simulink model "PWM_model_4screenshot"  (R2024b)
settings: Solver=odeN  StartTime=0.0  StopTime=35  MaxStep=5e-05  RelTol=0.001  EnableMultiTasking=on
InitFcn:
  | load bldcData
model workspace (MAT data in the model file):
  encoderResolution = 2000
  hallOffset = '0.5'
  indexOffset = 850
  polePairs = '4'
undefined symbols (not defined in the file or in its folder): Hecate_speed, Ts_motor
libraries: fl_lib x5, nesl_utility x2, ee_lib x1
settings Model: SimulationMode=accelerator  Creator=The MathWorks, Inc.  LastModifiedBy=andrea
settings SolverCC: ConsecutiveZCsStepRelTol=2.8421709430404e-13  AlgebraicLoopSolver=TrustRegion  AutoInsertRateTranBlk=on
settings DataIOCC: LimitDataPoints=on  SaveFormat=Array
settings OptimizationCC: DefaultParameterBehavior=Inlined  OptimizeBlockIOStorage=off  BufferReuse=off  GlobalBufferReuse=off  ExpressionFolding=off  ExpressionDepthLimit=2147483647  LocalBlockOutputs=off  ZeroExternalMemoryAtStartup=off  InitFltsAndDblsToZero=on  NoFixptDivByZeroProtection=on  EfficientFloat2IntCast=on  EfficientMapNaN2IntZero=off  LifeSpan=Inf  MaxStackSize=64  OptimizeDataStoreBuffers=off  BusAssignmentInplaceUpdate=off  EfficientTunableParamExpr=on
settings DebuggingCC: ReadBeforeWriteMsg=DisableAll  WriteAfterWriteMsg=DisableAll  WriteAfterReadMsg=DisableAll  CheckSSInitialOutputMsg=off  SignalResolutionControl=TryResolveAllWithWarning  SolverPrmCheckMsg=warning  InheritedTsInSrcMsg=none  MultiTaskDSMMsg=none  MultiTaskCondExecSysMsg=none  TasksWithSamePriorityMsg=none  SigSpecEnsureSampleTimeMsg=none  IntegerOverflowMsg=none  ParameterPrecisionLossMsg=none  FcnCallInpInsideContextMsg=warning  UnconnectedInputMsg=warning  UnconnectedOutputMsg=warning  UnconnectedLineMsg=warning  AllowSymbolicDim=off  StateNameClashWarn=warning  PregeneratedLibrarySubsystemCodeDiagnostic=none  SFUnexpectedBacktrackingDiag=warning  SFNoUnconditionalDefaultTransitionDiag=warning  SFExecutionAtInitializationDiag=none  IntegerSaturationMsg=none  ArithmeticOperatorsInVariantConditions=warning
settings HardwareCC: ProdBitPerChar=16  ProdBitPerInt=16  ProdBitPerPointer=32  ProdBitPerSizeT=32  ProdBitPerPtrDiffT=32  ProdLargestAtomicInteger=Integer  ProdLargestAtomicFloat=None  ProdWordSize=16  ProdLongLongMode=on  ProdHWDeviceType=Texas Instruments->C2000  TargetBitPerChar=16  TargetBitPerInt=16  TargetBitPerPointer=16  TargetLargestAtomicInteger=Integer  TargetIntDivRoundTo=Zero  TargetEndianess=LittleEndian  TargetWordSize=16  TargetHWDeviceType=TI C2000
settings ModelReferenceCC: EnableRefExpFcnMdlSchedulingChecks=on  PropagateSignalLabelsOutOfModel=off
settings SFSimCC: SimUseLocalCustomCode=off  MATLABDynamicMemAlloc=off
settings RTWCC: Description=Embedded Coder  SystemTargetFile=ert.tlc  TemplateMakefile=ert_default_tmf  GenerateReport=on  RTWUseLocalCustomCode=off  Toolchain=Texas Instruments Code Composer Studio (C2000)  IncludeHyperlinkInReport=on  LaunchReport=on  GenerateTraceInfo=on  GenerateTraceReport=on  GenerateTraceReportSl=on  GenerateTraceReportSf=on  GenerateTraceReportEml=on  GPUComputeCapability=3.5
settings CodeAppCC: IgnoreCustomStorageClasses=off  CustomSymbolStrType=$N$R$M  StateflowObjectComments=on  InternalIdentifier=Classic
settings ERTTargetCC: MultiwordLength=2048  InlinedParameterPlacement=Hierarchical  ERTCustomFileTemplate=example_file_process.tlc  ConvertIfToSwitch=off  SuppressUnreachableDefaultCases=off  MemSecPackage=tic2000demospkg  DynamicArrayContainerType=coder::array
settings ConfigComp: CovMetricSettings=dw  CovSaveCumulativeToWorkspaceVar=on  CovSaveSingleToWorkspaceVar=on  CovExternalEMLEnable=off  CovSFcnEnable=off

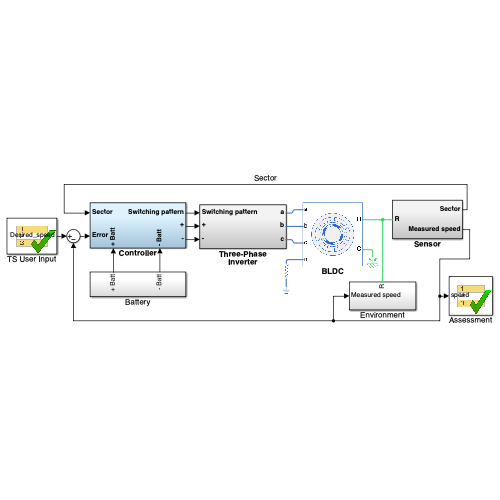
[thumbnail: Simulink's stored preview of the top-level diagram]
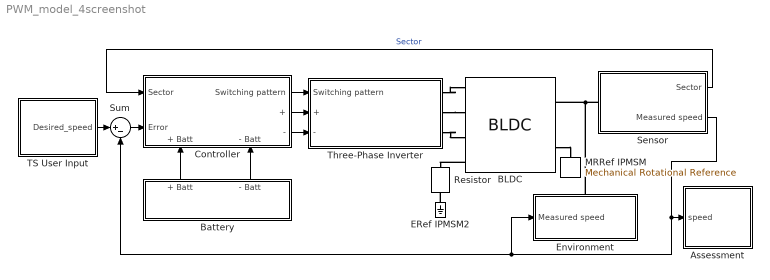
== system PWM_model_4screenshot ==
  Assessment : Test Sequence  TreatAsAtomicUnit=on
  BLDC : ee_lib/Electromechanical/Permanent Magnet/BLDC  port_option=ee.enum.threePhasePort.expanded  rotor_param=ee.enum.pmsm.backemf.trapezoidbackemf  pm_flux_linkage=0.18 Wb  theta_constant=120/23 deg  emf_max=20 V  w_meas=300 rpm  DphiDtheta_tab=[0, -.1528, -.1528, .1528, .1528, 0] Wb/rad  back_emf_tab=[0, -9.6, -9.6, 9.6, 9.6, 0] V  rotor_angle_tab=[0, 7.5, 22.5, 37.5, 52.5, 60] deg  nPolePairs=23  axes_param=ee.enum.rotorangle.daxis  winding_type=ee.enum.statorconnection.wye  stator_param=ee.enum.statorparam.LsLmMs  machine_param=ee.enum.dqparameterization.constant  Ld=0.00026 H  Lq=0.00026 H  idVec=[-200, 0, 200] A  iqVec=[-200, 0, 200] A  LdMatrix=0.00022 * ones(3, 3) H  LqMatrix=0.00022 * ones(3, 3) H  L0=0.00016 H  Ls=0.00026 H  Lm=0 H  Ms=0.00002 H  Rs=0.12 Ohm  zero_sequence=ee.enum.park.zerosequence.include  loss_param=ee.enum.ironloss.none  losses_oc=[0, 0, 0] W  losses_sc=[0, 0, 0] W  f_losses=60 Hz  Isc_losses=95 A  J=0 kg*m^2  lam=0.1 N*m/(rad/s)  i_d_specify=off  i_d_priority=None  i_d=0 A  i_d_nominal_specify=off  i_d_nominal_value=1  i_d_nominal_unit=A  i_q_specify=off  i_q_priority=None  i_q=0 A  i_q_nominal_specify=off  i_q_nominal_value=1  i_q_nominal_unit=A  torque_specify=off  torque_priority=None  torque=0 N*m  torque_nominal_specify=off  torque_nominal_value=1  torque_nominal_unit=N*m  angular_velocity_specify=off  angular_velocity_priority=High  angular_velocity=0 rpm  angular_velocity_nominal_specify=off  angular_velocity_nominal_value=1  angular_velocity_nominal_unit=rpm  angular_position_specify=off  angular_position_priority=High  angular_position=0 deg  angular_position_nominal_specify=off  angular_position_nominal_value=1  angular_position_nominal_unit=deg  alpha=3.93e-3 1/K  alpha_flux=-0.001 1/K  Tmeas=298.15 K  stator_thermal_mass=100 J/K  rotor_thermal_mass=200 J/K  Rm_percent_rotor=90  Rd_percent_rotor=30  temperatureA_specify=off  temperatureA_priority=High  temperatureA=25 degC  temperatureA_nominal_specify=off  temperatureA_nominal_value=1  temperatureA_nominal_unit=degC  temperatureB_specify=off  temperatureB_priority=High  temperatureB=25 degC  temperatureB_nominal_specify=off  temperatureB_nominal_value=1  temperatureB_nominal_unit=degC  temperatureC_specify=off  temperatureC_priority=High  temperatureC=25 degC  temperatureC_nominal_specify=off  temperatureC_nominal_value=1  temperatureC_nominal_unit=degC  temperatureR_specify=off  temperatureR_priority=High  temperatureR=25 degC  temperatureR_nominal_specify=off  temperatureR_nominal_value=1  temperatureR_nominal_unit=degC
      settings: InternalSimscapePortConfiguration="{\"Bottom\":[],\"Left\":[{\"id\":\"a\",\"label\":\"a\",\"type\":\"foundation.electrical.electrical\"},{\"id\":\"b\",\"label\":\"b\",\"type\":\"foundation.electrical.electrical\"},{\"id\":\"c\",\"label\":\"c\",\"type\":\"foundation.electrical.electrical\"},{\"id\":\"n\",\"label\":\"n\",\"type\":\"foundation.electrical.electrical\"}],\"Right\":[{\"id\":\"R\",\"label\":\"R\",\"type\":\"foundation.mechanical.rotational.rotational\"},{\"id\":\"C\",\"label\":\"C\",\"type\":\"foundation.mechanical.rotational.rotational\"}],\"Top\":[]}"
  Battery : Subsystem
      settings: PortSchema="{\"entries\":[{\"content\":{\"sides\":[{\"content\":{},\"type\":\"ConnectorPlacement.EquallySpacedRectSide\",\"uuid\":\"b9718aef-fc37-4786-bd99-1dccf9b07c4f\"},{\"content\":{\"side\":\"RIGHT\"},\"type\":\"ConnectorPlacement.EquallySpacedRectSide\",\"uuid\":\"5820c9b3-5480-4dfb-8619-e8171224d142\"},{\"content\":{\"connectorIds\":[\"Out1\",\"Out2\"],\"side\":\"TOP\"},\"type\":\"ConnectorPlacement.EquallySpacedRectSide\",\"uuid\":\"c449666b-5582-45da-b4a5-53b32c40c228\"}]},\"type\":\"ConnectorPlacement.EquallySpacedConnector\",\"uuid\":\"1a96bb2a-99ae-4235-9339-f0a559bfd98e\"}],\"packageUris\":[\"http://schema.mathworks.com/mf0/Connector/R2020b\"],\"version\":\"1.0\"}"
  Controller : Subsystem
      settings: PortSchema="{\"entries\":[{\"content\":{\"sides\":[{\"content\":{\"connectorIds\":[\"In1\",\"In2\"]},\"type\":\"ConnectorPlacement.EquallySpacedRectSide\",\"uuid\":\"2ab9d340-b50e-4422-9f4a-f0df7672da06\"},{\"content\":{\"connectorIds\":[\"Out1\",\"Out2\",\"Out3\"],\"side\":\"RIGHT\"},\"type\":\"ConnectorPlacement.EquallySpacedRectSide\",\"uuid\":\"8a4a8f23-4dad-4f8d-b073-fdebce0398f2\"},{\"content\":{\"side\":\"TOP\"},\"type\":\"ConnectorPlacement.EquallySpacedRectSide\",\"uuid\":\"b8c5a98d-225d-4655-b3bc-dd2e061911fb\"},{\"content\":{\"connectorIds\":[\"In3\",\"In4\"],\"side\":\"BOTTOM\"},\"type\":\"ConnectorPlacement.EquallySpacedRectSide\",\"uuid\":\"b2d3fee4-6eef-4d21-a73a-f8383ccb3ce8\"}]},\"type\":\"ConnectorPlacement.EquallySpacedConnector\",\"uuid\":\"adbcbcaa-ff3a-439a-b018-a3a47520a1df\"}],\"packageUris\":[\"http://schema.mathworks.com/mf0/Connector/R2020b\"],\"version\":\"1.0\"}"
  ERef IPMSM2 : fl_lib/Electrical/Electrical Elements/Electrical Reference
  Environment : Subsystem
      settings: PortSchema="{\"entries\":[{\"content\":{\"sides\":[{\"content\":{\"connectorIds\":[\"In1\"]},\"type\":\"ConnectorPlacement.EquallySpacedRectSide\",\"uuid\":\"b9718aef-fc37-4786-bd99-1dccf9b07c4f\"},{\"content\":{\"side\":\"RIGHT\"},\"type\":\"ConnectorPlacement.EquallySpacedRectSide\",\"uuid\":\"5820c9b3-5480-4dfb-8619-e8171224d142\"},{\"content\":{\"connectorIds\":[\"LConn1\"],\"side\":\"TOP\"},\"type\":\"ConnectorPlacement.EquallySpacedRectSide\",\"uuid\":\"c449666b-5582-45da-b4a5-53b32c40c228\"}]},\"type\":\"ConnectorPlacement.EquallySpacedConnector\",\"uuid\":\"1a96bb2a-99ae-4235-9339-f0a559bfd98e\"}],\"packageUris\":[\"http://schema.mathworks.com/mf0/Connector/R2020b\"],\"version\":\"1.0\"}"
  MRRef IPMSM : fl_lib/Mechanical/Rotational Elements/Mechanical Rotational Reference
  Resistor : fl_lib/Electrical/Electrical Elements/Resistor  R=1e9 Ohm  i_specify=off  i_priority=None  i=0 A  i_nominal_specify=off  i_nominal_value=1  i_nominal_unit=A  v_specify=off  v_priority=None  v=0 V  v_nominal_specify=off  v_nominal_value=1  v_nominal_unit=V
  Sensor : Subsystem
  Sum : Sum  Inputs=|+-
  TS User Input : Test Sequence  TreatAsAtomicUnit=on
  Three-Phase Inverter : Subsystem
  wires:
  Sensor/1(Sector) -> Controller/1(Sector)  "Sector"
  Sum/1 -> Controller/2(Error)
  TS User Input/1(Desired_speed) -> Sum/1
  Controller/1(Switching pattern) -> Three-Phase Inverter/1(Switching pattern)
  Battery/1(+ Batt) -> Controller/3(+ Batt)
  Battery/2(- Batt) -> Controller/4(- Batt)
  Controller/2(+) -> Three-Phase Inverter/2(+)
  Controller/3(-) -> Three-Phase Inverter/3(-)
  Sensor/2(Measured speed) -> Environment/1(Measured speed), Sum/2, Assessment/1(speed)
  connections:
  ERef IPMSM2/LConn1 -- Resistor/RConn1
  BLDC/LConn4 -- Resistor/LConn1
  Sensor/LConn1 -- Environment/LConn1 -- BLDC/RConn1
  BLDC/RConn2 -- MRRef IPMSM/LConn1
  Three-Phase Inverter/RConn1 -- BLDC/LConn1
  Three-Phase Inverter/RConn2 -- BLDC/LConn2
  Three-Phase Inverter/RConn3 -- BLDC/LConn3

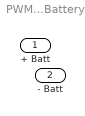
== system PWM_model_4screenshot/Battery ==
  + Batt : Outport
  - Batt : Outport  Port=2

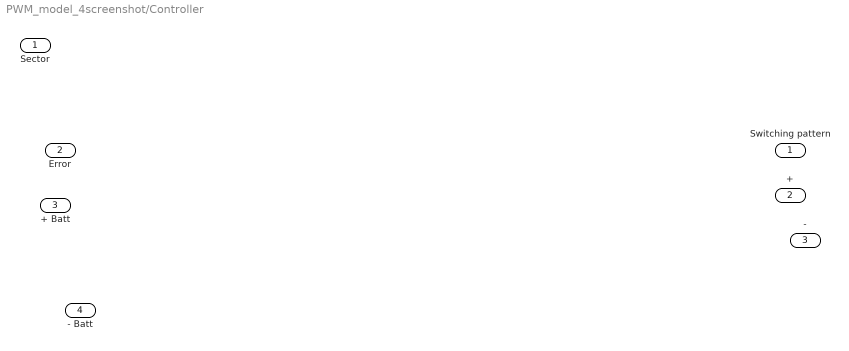
== system PWM_model_4screenshot/Controller ==
  Sector : Inport
  Error : Inport  Port=2
  + Batt : Inport  Port=3
  - Batt : Inport  Port=4
  Switching pattern : Outport
  + : Outport  Port=2
  - : Outport  Port=3

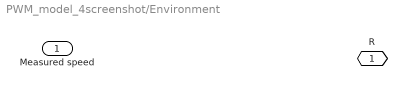
== system PWM_model_4screenshot/Environment ==
  Measured speed : Inport
  R : PMIOPort  Side=Left

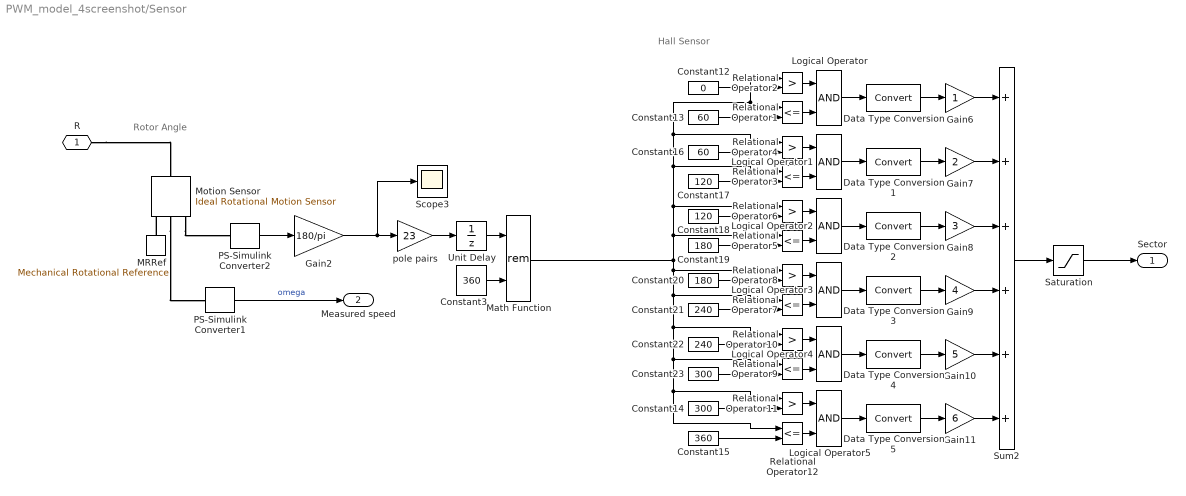
== system PWM_model_4screenshot/Sensor ==
  note: Rotor Angle
  note: Hall Sensor
  Constant12 : Constant  Value=0
  Constant13 : Constant  Value=60
  Constant14 : Constant  Value=300
  Constant15 : Constant  Value=360
  Constant16 : Constant  Value=60
  Constant17 : Constant  Value=120
  Constant18 : Constant  Value=120
  Constant19 : Constant  Value=180
  Constant20 : Constant  Value=180
  Constant21 : Constant  Value=240
  Constant22 : Constant  Value=240
  Constant23 : Constant  Value=300
  Constant3 : Constant  Value=360
  Data Type Conversion{,1..5} (6 alike) : DataTypeConversion
  Gain10 : Gain  Gain=5  SaturateOnIntegerOverflow=on  OutDataTypeStr=Inherit: Same as input  ParamDataTypeStr=Inherit: Same as input
  Gain11 : Gain  Gain=6  SaturateOnIntegerOverflow=on  OutDataTypeStr=Inherit: Same as input  ParamDataTypeStr=Inherit: Same as input
  Gain2 : Gain  Gain=180/pi
  Gain6 : Gain  SaturateOnIntegerOverflow=on  OutDataTypeStr=Inherit: Same as input  ParamDataTypeStr=Inherit: Same as input
  Gain7 : Gain  Gain=2  SaturateOnIntegerOverflow=on  OutDataTypeStr=Inherit: Same as input  ParamDataTypeStr=Inherit: Same as input
  Gain8 : Gain  Gain=3  SaturateOnIntegerOverflow=on  OutDataTypeStr=Inherit: Same as input  ParamDataTypeStr=Inherit: Same as input
  Gain9 : Gain  Gain=4  SaturateOnIntegerOverflow=on  OutDataTypeStr=Inherit: Same as input  ParamDataTypeStr=Inherit: Same as input
  Logical Operator{,1..5} (6 alike) : Logic
  MRRef : fl_lib/Mechanical/Rotational Elements/Mechanical Rotational Reference
  Math Function : Math  Operator=rem  SignedPower=on
  Motion Sensor : fl_lib/Mechanical/Mechanical Sensors/Ideal Rotational Motion Sensor  reference=foundation.enum.MeasurementReference.difference  acceleration_port=false  velocity_port=true  position_port=true  wrap_angle=false  offset=0 deg
  PS-Simulink Converter1 : nesl_utility/PS-Simulink Converter  PhysicalDomain=network_engine_domain  SubClassName=ps_output  LeftPortType=input  RightPortType=output  PseudoPeriodic=off  Frequencies=[]  VectorFormat=1-D array  Unit=rpm  AffineConversion=off
  PS-Simulink Converter2 : nesl_utility/PS-Simulink Converter  PhysicalDomain=network_engine_domain  SubClassName=ps_output  LeftPortType=input  RightPortType=output  PseudoPeriodic=off  Frequencies=[]  VectorFormat=1-D array  Unit=rad  AffineConversion=off
  Relational Operator{1,3,5,7,9,12} (6 alike) : RelationalOperator  Operator=<=
  Relational Operator{2,4,6,8,10..11} (6 alike) : RelationalOperator  Operator=>
  Saturation : Saturate  UpperLimit=6  LowerLimit=1
  Scope3 : Scope
  Sum2 : Sum  Inputs=++++++  InputSameDT=on  SaturateOnIntegerOverflow=on  OutDataTypeStr=Inherit: Same as first input
  Unit Delay : UnitDelay  SampleTime=Ts_motor  HasFrameUpgradeWarning=on
  pole pairs : Gain  Gain=23
  R : PMIOPort  Side=Left
  Sector : Outport
  Measured speed : Outport  Port=2
  wires:
  Saturation/1 -> Sector/1
  Math Function/1 -> Relational Operator2/1, Relational Operator1/1, Relational Operator4/1, Relational Operator3/1, Relational Operator6/1, Relational Operator5/1, Relational Operator12/1, Relational Operator11/1, Relational Operator9/1, Relational Operator10/1, Relational Operator7/1, Relational Operator8/1
  Data Type Conversion5/1 -> Gain11/1
  Data Type Conversion4/1 -> Gain10/1
  Data Type Conversion3/1 -> Gain9/1
  Data Type Conversion2/1 -> Gain8/1
  Data Type Conversion1/1 -> Gain7/1
  Data Type Conversion/1 -> Gain6/1
  Relational Operator2/1 -> Logical Operator/1
  Relational Operator1/1 -> Logical Operator/2
  Logical Operator/1 -> Data Type Conversion/1
  Constant12/1 -> Relational Operator2/2
  Constant13/1 -> Relational Operator1/2
  Relational Operator4/1 -> Logical Operator1/1
  Relational Operator3/1 -> Logical Operator1/2
  Logical Operator1/1 -> Data Type Conversion1/1
  Constant16/1 -> Relational Operator4/2
  Constant17/1 -> Relational Operator3/2
  Relational Operator6/1 -> Logical Operator2/1
  Relational Operator5/1 -> Logical Operator2/2
  Logical Operator2/1 -> Data Type Conversion2/1
  Constant18/1 -> Relational Operator6/2
  Constant19/1 -> Relational Operator5/2
  Relational Operator8/1 -> Logical Operator3/1
  Relational Operator7/1 -> Logical Operator3/2
  Logical Operator3/1 -> Data Type Conversion3/1
  Constant20/1 -> Relational Operator8/2
  Constant21/1 -> Relational Operator7/2
  Relational Operator10/1 -> Logical Operator4/1
  Relational Operator9/1 -> Logical Operator4/2
  Logical Operator4/1 -> Data Type Conversion4/1
  Constant22/1 -> Relational Operator10/2
  Constant23/1 -> Relational Operator9/2
  Relational Operator11/1 -> Logical Operator5/1
  Relational Operator12/1 -> Logical Operator5/2
  Logical Operator5/1 -> Data Type Conversion5/1
  Constant14/1 -> Relational Operator11/2
  Constant15/1 -> Relational Operator12/2
  Gain6/1 -> Sum2/1
  Gain7/1 -> Sum2/2
  Gain8/1 -> Sum2/3
  Gain9/1 -> Sum2/4
  Gain10/1 -> Sum2/5
  Gain11/1 -> Sum2/6
  Sum2/1 -> Saturation/1
  PS-Simulink Converter2/1 -> Gain2/1
  Gain2/1 -> Scope3/1, pole pairs/1
  Constant3/1 -> Math Function/2
  pole pairs/1 -> Unit Delay/1
  Unit Delay/1 -> Math Function/1
  PS-Simulink Converter1/1 -> Measured speed/1  "omega"
  connections:
  Motion Sensor/RConn3 -- PS-Simulink Converter2/LConn1
  MRRef/LConn1 -- Motion Sensor/RConn1
  Motion Sensor/RConn2 -- PS-Simulink Converter1/LConn1
  R/RConn1 -- Motion Sensor/LConn1

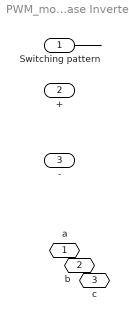
== system PWM_model_4screenshot/Three-Phase Inverter ==
  Switching pattern : Inport
  + : Inport  Port=2
  - : Inport  Port=3
  a : PMIOPort  Side=Right
  b : PMIOPort  Port=2  Side=Right
  c : PMIOPort  Port=3  Side=Right
  wires:
  Switching pattern/1 -> ?

== stateflow chart PWM_model_4screenshot/TS User Input ==
  state Grafico_Scalino_1
    state step_1
      speed = 0;
    state step_2
      speed = Hecate_speed;
    (default) -> Grafico_Scalino_1.step_1
    Grafico_Scalino_1.step_1 -> Grafico_Scalino_1.step_2 : [
        | after(1,'sec')
        | ]
    Grafico_Scalino_1.step_2 -> Grafico_Scalino_1.step_1 : [
        | after(4,'sec')
        | ]
  state Grafico_Scalino_2
    state step_1
      speed = 85;
    state step_2
      speed = Hecate_speed;
    (default) -> Grafico_Scalino_2.step_1
    Grafico_Scalino_2.step_1 -> Grafico_Scalino_2.step_2 : [
        | after(1,'sec')
        | ]
    Grafico_Scalino_2.step_2 -> Grafico_Scalino_2.step_1 : [
        | after(4,'sec')
        | ]
  state Grafico_Scalino_3
    state step_1
      speed = 130;
    state step_2
      speed = Hecate_speed;
    (default) -> Grafico_Scalino_3.step_1
    Grafico_Scalino_3.step_1 -> Grafico_Scalino_3.step_2 : [
        | after(1,'sec')
        | ]
    Grafico_Scalino_3.step_2 -> Grafico_Scalino_3.step_1 : [
        | after(4,'sec')
        | ]
  state Grafico_DoppioTronco_1
    state step_1
      getSimulationTime()
      speed = 0 + (Hecate_speed - 0) / (5 - 0) * getSimulationTime();
    state step_2
      speed = Hecate_speed;
    state step_3
      speed = Hecate_speed + (0 - Hecate_speed) / (15 - 10) * (getSimulationTime - 10);
    state step_4
      speed = 0;
    state step_5
      speed = 0 + (Hecate_speed - 0) / (5 - 0) * (getSimulationTime() - 20);
    state step_6
      speed = Hecate_speed;
    state step_7
      speed = Hecate_speed + (0 - Hecate_speed) / (15 - 10) * (getSimulationTime - 30);
    (default) -> Grafico_DoppioTronco_1.step_1
    Grafico_DoppioTronco_1.step_1 -> Grafico_DoppioTronco_1.step_2 : [
        | after(5, 'sec')
        | ]
    Grafico_DoppioTronco_1.step_2 -> Grafico_DoppioTronco_1.step_3 : [
        | after(5, 'sec')
        | ]
    Grafico_DoppioTronco_1.step_3 -> Grafico_DoppioTronco_1.step_4 : [
        | after(5, 'sec')
        | ]
    Grafico_DoppioTronco_1.step_4 -> Grafico_DoppioTronco_1.step_5 : [
        | after(5, 'sec')
        | ]
    Grafico_DoppioTronco_1.step_5 -> Grafico_DoppioTronco_1.step_6 : [
        | after(5, 'sec')
        | ]
    Grafico_DoppioTronco_1.step_6 -> Grafico_DoppioTronco_1.step_7 : [
        | after(5, 'sec')
        | ]
  state Grafico_DoppioTronco_2
    state step_1
      getSimulationTime()
      speed = 85 + (Hecate_speed - 85) / (5 - 0) * getSimulationTime();
    state step_2
      speed = Hecate_speed;
    state step_3
      speed = Hecate_speed + (85 - Hecate_speed) / (15 - 10) * (getSimulationTime - 10);
    state step_4
      speed = 85;
    state step_5
      speed = 85 + (Hecate_speed - 85) / (5 - 0) * (getSimulationTime() - 20);
    state step_6
      speed = Hecate_speed;
    state step_7
      speed = Hecate_speed + (85 - Hecate_speed) / (15 - 10) * (getSimulationTime - 30);
    (default) -> Grafico_DoppioTronco_2.step_1
    Grafico_DoppioTronco_2.step_1 -> Grafico_DoppioTronco_2.step_2 : [
        | after(5, 'sec')
        | ]
    Grafico_DoppioTronco_2.step_2 -> Grafico_DoppioTronco_2.step_3 : [
        | after(5, 'sec')
        | ]
    Grafico_DoppioTronco_2.step_3 -> Grafico_DoppioTronco_2.step_4 : [
        | after(5, 'sec')
        | ]
    Grafico_DoppioTronco_2.step_4 -> Grafico_DoppioTronco_2.step_5 : [
        | after(5, 'sec')
        | ]
    Grafico_DoppioTronco_2.step_5 -> Grafico_DoppioTronco_2.step_6 : [
        | after(5, 'sec')
        | ]
    Grafico_DoppioTronco_2.step_6 -> Grafico_DoppioTronco_2.step_7 : [
        | after(5, 'sec')
        | ]
  state Grafico_DoppioTronco_3
    state step_1
      getSimulationTime()
      speed = 130 + (Hecate_speed - 130) / (5 - 0) * getSimulationTime();
    state step_2
      speed = Hecate_speed;
    state step_3
      speed = Hecate_speed + (130 - Hecate_speed) / (15 - 10) * (getSimulationTime - 10);
    state step_4
      speed = 130;
    state step_5
      speed = 130 + (Hecate_speed - 130) / (5 - 0) * (getSimulationTime() - 20);
    state step_6
      speed = Hecate_speed;
    state step_7
      speed = Hecate_speed + (130 - Hecate_speed) / (15 - 10) * (getSimulationTime - 30);
    (default) -> Grafico_DoppioTronco_3.step_1
    Grafico_DoppioTronco_3.step_1 -> Grafico_DoppioTronco_3.step_2 : [
        | after(5, 'sec')
        | ]
    Grafico_DoppioTronco_3.step_2 -> Grafico_DoppioTronco_3.step_3 : [
        | after(5, 'sec')
        | ]
    Grafico_DoppioTronco_3.step_3 -> Grafico_DoppioTronco_3.step_4 : [
        | after(5, 'sec')
        | ]
    Grafico_DoppioTronco_3.step_4 -> Grafico_DoppioTronco_3.step_5 : [
        | after(5, 'sec')
        | ]
    Grafico_DoppioTronco_3.step_5 -> Grafico_DoppioTronco_3.step_6 : [
        | after(5, 'sec')
        | ]
    Grafico_DoppioTronco_3.step_6 -> Grafico_DoppioTronco_3.step_7 : [
        | after(5, 'sec')
        | ]
  (default) -> Grafico_Scalino_1 [order 1] : [Active_Scenario_Index == 1]
  (default) -> Grafico_Scalino_2 [order 2] : [Active_Scenario_Index == 2]
  (default) -> Grafico_Scalino_3 [order 3] : [Active_Scenario_Index == 3]
  (default) -> Grafico_DoppioTronco_1 [order 4] : [Active_Scenario_Index == 4]
  (default) -> Grafico_DoppioTronco_2 [order 5] : [Active_Scenario_Index == 5]
  (default) -> Grafico_DoppioTronco_3 [order 6] : {assert(Active_Scenario_Index == 6,'The value of Scenario Parameter ''Active_Scenario_Index'' is not valid. Use the index of the scenario to specify it.')}
  data: Desired_speed output; Active_Scenario_Index parameter =1; Hecate_speed parameter

== stateflow chart PWM_model_4screenshot/Assessment ==
  state SpeedLimit_0
    state step_1
    state step_2
      verify(speed >= 0.0001);
    (default) -> SpeedLimit_0.step_1
    SpeedLimit_0.step_1 -> step_2 : [
        | after(2, 'sec')
        | ]
  state SpeedLimit_170
    state Speed_Hecate
      verify(speed <=  170);
    (default) -> SpeedLimit_170.Speed_Hecate
  state SpeedLimit_HS
    state step_1
      % Initial and Final Waiting Period
    state Speed_Hecate
      verify(speed <= (Hecate_speed + 1));
    state step_3
      % Midpoint Waiting Period
    state Speed_Hecate_1
      verify(speed <= (Hecate_speed + 1));
    (default) -> SpeedLimit_HS.step_1
    (junction 384) -> SpeedLimit_HS.step_1
    SpeedLimit_HS.step_1 -> SpeedLimit_HS.Speed_Hecate : [
        | after(6, 'sec')
        | ]
    SpeedLimit_HS.Speed_Hecate -> step_3 : [
        | after(4, 'sec')
        | ]
    step_3 -> Speed_Hecate_1 : [
        | after(16, 'sec')
        | ]
    Speed_Hecate_1 -> (junction 386) : [
        | after(4, 'sec')
        | ]
    (junction 386) -> (junction 384)
  state SpeedLimit_HS_subtest
    state step_1
    state Speed_Hecate
      verify(speed <= (Hecate_speed + 1));
    (default) -> SpeedLimit_HS_subtest.step_1
    SpeedLimit_HS_subtest.step_1 -> SpeedLimit_HS_subtest.Speed_Hecate : [
        | after(26, 'sec')
        | ]
    SpeedLimit_HS_subtest.Speed_Hecate -> SpeedLimit_HS_subtest.step_1 : [
        | after(4, 'sec')
        | ]
  (default) -> SpeedLimit_0 [order 1] : [Active_Scenario_Index == 1]
  (default) -> SpeedLimit_170 [order 2] : [Active_Scenario_Index == 2]
  (default) -> SpeedLimit_HS [order 3] : [Active_Scenario_Index == 3]
  (default) -> SpeedLimit_HS_subtest [order 4] : {assert(Active_Scenario_Index == 4,'The value of Scenario Parameter ''Active_Scenario_Index'' is not valid. Use the index of the scenario to specify it.')}
  data: speed input; Active_Scenario_Index parameter =1; speed_at_5_5 local; speed_at_9 local; Hecate_speed parameter
